simulink model "Microgrid_uniTLM_server"  (R2025b)
settings: Solver=ode3  StartTime=0.0  StopTime=1  FixedStep=params.sampleTime  RelTol=1e-3
InitFcn:
  | unitlmModelFile = get_param(bdroot, 'FileName');
  | if ~isempty(unitlmModelFile), addpath(fileparts(unitlmModelFile)); end
  | initialize_unitlm_microgrid();
  | clear unitlmModelFile
StartFcn:
  | unitlmModelFile = get_param(bdroot, 'FileName'); if ~isempty(unitlmModelFile), addpath(fileparts(unitlmModelFile)); end; try, if exist('unitlm_timing_probe', 'file') == 2, unitlm_timing_probe('start', 'server', bdroot); else, warning('uniTLM:TimingProbeNotFound', 'unitlm_timing_probe.m not found on MATLAB path; timing probe disabled.'); end; catch unitlmTimingError, warning('uniTLM:TimingProbeFailed', 'unitlm_timing_probe failed: %s', unitlmTimingError.message); end; clear unitlmModelFile
StopFcn:
  | unitlmModelFile = get_param(bdroot, 'FileName'); if ~isempty(unitlmModelFile), addpath(fileparts(unitlmModelFile)); end; try, if exist('unitlm_timing_probe', 'file') == 2, unitlm_timing_probe('stop', 'server', bdroot); else, warning('uniTLM:TimingProbeNotFound', 'unitlm_timing_probe.m not found on MATLAB path; timing probe disabled.'); end; catch unitlmTimingError, warning('uniTLM:TimingProbeFailed', 'unitlm_timing_probe failed: %s', unitlmTimingError.message); end; clear unitlmModelFile
  | %% StopFcn: save TLM server-side results
  | 
  | modelName = bdroot;
  | modelFile = get_param(modelName, 'FileName');
  | 
  | if isempty(modelFile)
  |     modelDir = pwd;
  | else
  |     modelDir = fileparts(modelFile);
  | end
  | 
  | resultDir = fullfile(modelDir, 'result');
  | 
  | if ~exist(resultDir, 'dir')
  |     mkdir(resultDir);
  | end
  | 
  | % Server-side workspace variables
  | variableNames = {
  |     'server_voltage'
  |     'server_current'
  |     'server_PQ'
  | };
  | 
  | serverTLMData = struct();
  | 
  | for k = 1:numel(variableNames)
  | 
  |     originalName = variableNames{k};
  |     saveName = [originalName, '_TLM'];
  | 
  |     if evalin('base', sprintf('exist(''%s'', ''var'')', originalName))
  |         serverTLMData.(saveName) = evalin('base', originalName);
  |     else
  |         warning( ...
  |             'StopFcn:MissingVariable', ...
  |             'Variable "%s" was not found in the base workspace.', ...
  |             originalName);
  |     end
  | end
  | 
  | % Save to result/server_TLM.mat
  | saveFile = fullfile(resultDir, 'server_TLM.mat');
  | save(saveFile, '-struct', 'serverTLMData');
  | 
  | fprintf('TLM server-side results saved to:\n%s\n', saveFile);
values from neighbouring files (symbols this model uses):
  Cf = Cf_pu*Cb    [initialize_unitlm_microgrid.m]
  f = logspace(log10(fMin), log10(fMax), nFrequency).'    [fit_non_heaviside_line_rational.m]    (also in initialize_unitlm_microgrid.m = 50)
  fsw1 = 10e3    (= 10000)    [initialize_unitlm_microgrid.m]
  Ip = 2*P/(3*Vp)    [initialize_unitlm_microgrid.m]
  L1 = L1_pu*Lb    [initialize_unitlm_microgrid.m]
  L2 = L2_pu*Lb    [initialize_unitlm_microgrid.m]
  L3 = L3_pu*Lb    [initialize_unitlm_microgrid.m]
  L4 = L4_pu*Lb    [initialize_unitlm_microgrid.m]
  Lc = Lc_pu*Lb    [initialize_unitlm_microgrid.m]
  Lf2 = Lf2_pu*Lb    [initialize_unitlm_microgrid.m]
  line_aHr = interface.line_aHr    [initialise_optimised_tlm_interface.m]    (also in initialize_unitlm_microgrid.m = real(line_aHr))
  line_aZc = interface.line_aZc    [initialise_optimised_tlm_interface.m]    (also in initialize_unitlm_microgrid.m = real(line_aZc))
  line_bHr = interface.line_bHr    [initialise_optimised_tlm_interface.m]    (also in initialize_unitlm_microgrid.m = real(line_bHr))
  line_bZc = interface.line_bZc    [initialise_optimised_tlm_interface.m]    (also in initialize_unitlm_microgrid.m = real(line_bZc))
  P = 5e6    (= 5000000)    [initialize_unitlm_microgrid.m]
  params = varargin{1}    [Client_co.m]    (also in Client_co_TLM.m; Server_co.m; Server_co_TLM.m; initialise_optimised_tlm_interface.m = config.cosimParams)
  R1 = R1_pu*Zb    [initialize_unitlm_microgrid.m]
  R2 = R2_pu*Zb    [initialize_unitlm_microgrid.m]
  R3 = R3_pu*Zb    [initialize_unitlm_microgrid.m]
  R4 = R4_pu*Zb    [initialize_unitlm_microgrid.m]
  Rdamp = Rf    [initialize_unitlm_microgrid.m]
  Rf = Rf_pu*Zb    [initialize_unitlm_microgrid.m]
  Rload1 = Vp/Ip    [initialize_unitlm_microgrid.m]
  Rload2 = Vp/Ip    [initialize_unitlm_microgrid.m]
  Rload3 = Vp/Ip    [initialize_unitlm_microgrid.m]
  Rv_pu = 0.1    [initialize_unitlm_microgrid.m]
  Sxfmr = 6.3e6    (= 6300000)    [initialize_unitlm_microgrid.m]
  Vac = sqrt(2)*Vline/sqrt(3)    [initialize_unitlm_microgrid.m]
  Vhv = 66e3    (= 66000)    [initialize_unitlm_microgrid.m]
  Vline = 690    [initialize_unitlm_microgrid.m]
  Vp = Vac    [initialize_unitlm_microgrid.m]
  Wb = 2*pi*f    (= 314.159265359)    [initialize_unitlm_microgrid.m]
  Xv_pu = 0.3    [initialize_unitlm_microgrid.m]
  Z_inf = interface.Z_inf    [initialise_optimised_tlm_interface.m]    (also in initialize_unitlm_microgrid.m = line_Zinf)
undefined symbols (not defined in the file or in its folder): DiscIntNeverNeededParam, DPL, dspblkCoreblockFVToolHelper, gcbh, Lline1
libraries: spsThreePhaseSeriesRLCBranchLib x14, spsControlledVoltageSourceLib x12, spsThreePhaseVIMeasurementLib x7, spsabctodq0Lib x6, slpidlib x4, spsThreePhaseBreakerLib x3, SimplusGT x3, spsThreePhaseTransformerTwoWindingsLib x3, spsPower3phInstantaneousLib x2, spsdq0toabcLib x2, spsDistributedParametersLineLib x1, simulink x1
(part 1 of 2)
settings Model: Creator=L  LastModifiedBy=Zhai Xinjie
settings DataIOCC: LimitDataPoints=on  SaveFormat=Array  ReturnWorkspaceOutputs=off
settings OptimizationCC: ReuseModelBlockBuffer=off  LifeSpan=inf
settings DebuggingCC: UnderspecifiedInitializationDetection=Classic  MergeDetectMultiDrivingBlocksExec=none  SolverPrmCheckMsg=warning  UnconnectedInputMsg=warning  UnconnectedOutputMsg=warning  UnconnectedLineMsg=warning  StateNameClashWarn=warning  SFUnexpectedBacktrackingDiag=warning  SFNoUnconditionalDefaultTransitionDiag=warning  SFExecutionAtInitializationDiag=none  ArithmeticOperatorsInVariantConditions=warning
settings HardwareCC: ProdBitPerPointer=32.0  ProdBitPerSizeT=32.0  ProdBitPerPtrDiffT=32.0  ProdLargestAtomicFloat=None  ProdIntDivRoundTo=Undefined  ProdEndianess=Unspecified  ProdWordSize=32.0  ProdHWDeviceType=32-bit Generic
settings ModelReferenceCC: EnableRefExpFcnMdlSchedulingChecks=on  PropagateSignalLabelsOutOfModel=off
settings SFSimCC: SimUseLocalCustomCode=off  CustomCodeUndefinedFunction=UseInterfaceOnly
settings RTWCC: RTWUseLocalCustomCode=off  GPUComputeCapability=3.5  DLArmComputeVersion=19.05
settings CodeAppCC: StateflowObjectComments=on
settings GRTTargetCC: TargetLangStandard=C89/C90 (ANSI)
settings ConfigComp: CovMetricSettings=dw  CovSaveCumulativeToWorkspaceVar=on  CovSaveSingleToWorkspaceVar=on  CovExternalEMLEnable=off
settings SimscapeCC: SimscapeNormalizeSystem=off

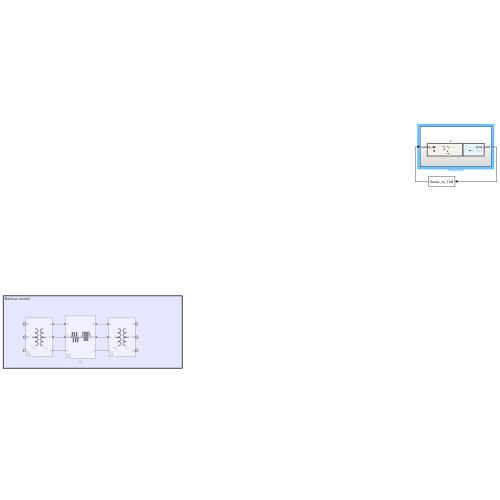
[thumbnail: Simulink's stored preview of the top-level diagram]
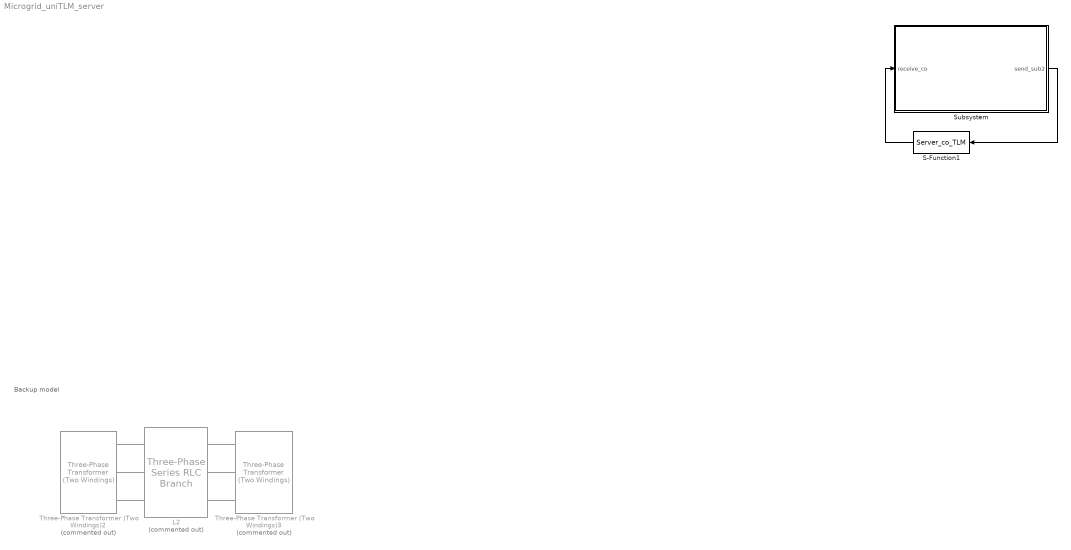
== system Microgrid_uniTLM_server ==
  note: Backup model
  L2 : spsThreePhaseSeriesRLCBranchLib/Three-Phase Series RLC Branch  Commented=on  LConnTagsString=A|B|C  RConnTagsString=A|B|C  BranchType=RL  Resistance=R2  Inductance=L2  Capacitance=1e-6  Measurements=None
  S-Function1 : S-Function  FunctionName=Server_co_TLM  SFunctionDeploymentMode=off  EnableBusSupport=off
  Subsystem : Subsystem
  Three-Phase Transformer (Two Windings)2 : spsThreePhaseTransformerTwoWindingsLib/Three-Phase Transformer (Two Windings)  Commented=on  Winding1Connection=Yg  Winding2Connection=Yg  CoreType=Three single-phase transformers  SetSaturation=off  Hysteresis=off  DataFile='hysteresis'  SetInitialFlux=off  Measurements=None  UNITS=pu  NominalPower=[ 250e6 , 50 ]  Winding1=[ 380e3 , 0.002 , 0.08 ]  Winding2=[ 33e3 , 0.002 , 0.08 ]  Rm=500  Lm=500  L0=0.5  Saturation=[ 0,0 ; 0.0024,1.2 ; 1.0,1.52 ]  InitialFluxes=[ 0.8 , -0.8 , 0.7 ]  BreakLoop=off  DiscreteSolver=Trapezoidal iterative  DataType=off  TransfoNumber=1
  Three-Phase Transformer (Two Windings)3 : spsThreePhaseTransformerTwoWindingsLib/Three-Phase Transformer (Two Windings)  Commented=on  Winding1Connection=Yg  Winding2Connection=Yg  CoreType=Three single-phase transformers  SetSaturation=off  Hysteresis=off  DataFile='hysteresis'  SetInitialFlux=off  Measurements=None  UNITS=pu  NominalPower=[ 250e6 , 50 ]  Winding1=[ 33e3 , 0.002 , 0.08 ]  Winding2=[ 380 , 0.002 , 0.08 ]  Rm=500  Lm=500  L0=0.5  Saturation=[ 0,0 ; 0.0024,1.2 ; 1.0,1.52 ]  InitialFluxes=[ 0.8 , -0.8 , 0.7 ]  BreakLoop=off  DiscreteSolver=Trapezoidal iterative  DataType=off  TransfoNumber=1
  wires:
  S-Function1/1 -> Subsystem/1(receive_co)
  Subsystem/1(send_sub2) -> S-Function1/1
  connections:
  Three-Phase Transformer (Two Windings)3/RConn1 -- L2/RConn1
  Three-Phase Transformer (Two Windings)3/RConn2 -- L2/RConn2
  Three-Phase Transformer (Two Windings)3/RConn3 -- L2/RConn3
  Three-Phase Transformer (Two Windings)2/RConn1 -- L2/LConn1
  Three-Phase Transformer (Two Windings)2/RConn2 -- L2/LConn2
  Three-Phase Transformer (Two Windings)2/RConn3 -- L2/LConn3

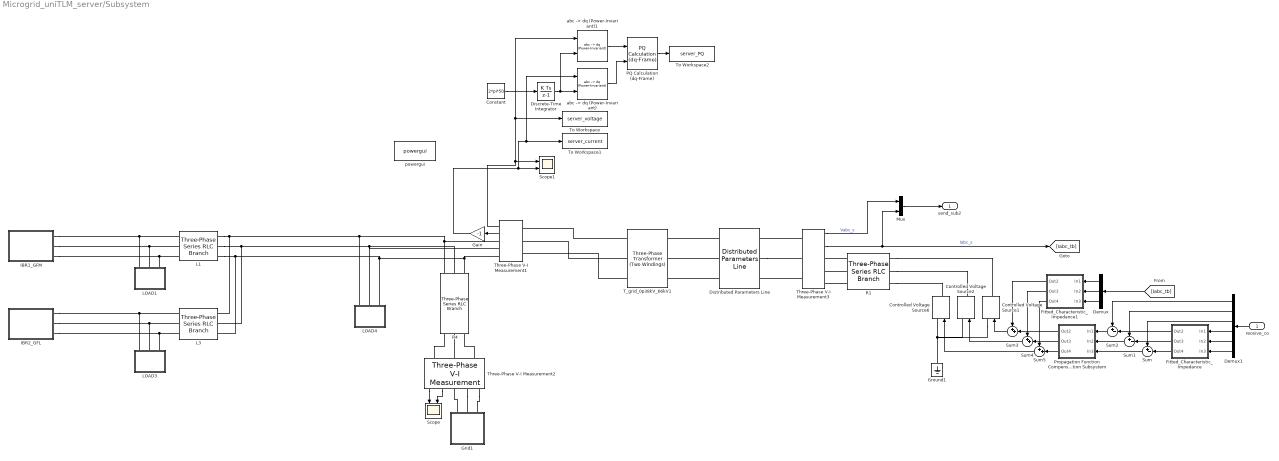
== system Microgrid_uniTLM_server/Subsystem ==
  receive_co : Inport
  Constant : Constant  Value=2*pi*50
  Controlled Voltage Source1 : spsControlledVoltageSourceLib/Controlled Voltage Source  Initialize=on  Source_Type=AC  Amplitude=0  Phase=0  Frequency=0  Measurements=None
  Controlled Voltage Source2 : spsControlledVoltageSourceLib/Controlled Voltage Source  Initialize=on  Source_Type=AC  Amplitude=0  Phase=0  Frequency=0  Measurements=None
  Controlled Voltage Source6 : spsControlledVoltageSourceLib/Controlled Voltage Source  Initialize=on  Source_Type=AC  Amplitude=0  Phase=0  Frequency=0  Measurements=None
  Demux : Demux  Outputs=3
  Demux1 : Demux  Outputs=6
  Discrete-Time Integrator : DiscreteIntegrator  SampleTime=-1  ICPrevOutput=DiscIntNeverNeededParam  ICPrevScaledInput=DiscIntNeverNeededParam
  Distributed Parameters Line : spsDistributedParametersLineLib/Distributed Parameters Line  Phases=3  Length=DPL.length  Frequency=DPL.freq  Resistance=DPL.R  Inductance=DPL.L  Capacitance=DPL.C  x1=[-0.0001175 0 0 0;-0.000117 0 0 0;-0.0001165 0 0 0;-0.000116 0 0 0;-0.0001155 0 0 0;-0.000115 0 0 0;-0.0001145 0 0 0;-0.000114 0 0 0;-0.0001135 0 0 0;-0.000113 0 0 0;-0.0001125 0 0 0;-0.000112 0 0 0;-0.0001115 0 0 0;-0.000111 0 0 0;-0.0001105 0 0 0;-0.00011 0 0 0;-0.0001095 0 0 0;-0.000109 0 0 0;-0.0001085 0 0 0;-0.000108 0 0 0;-0.0001075 0 0 0;-0.000107 0 0 0;-0.0001065 0 0 0;-0.000106 0 0 0;-0.0001055 0 0 0;-0.000105 0 0 0;-0.0001045 0 0 0;-0.000104 0 0 0;-0.0001035 0 0 0;-0.000103 0 0 0;-0.0001025 0 0 0;-0.000102 0 0 0;-0.0001015 0 0 0;-0.000101 0 0 0;-0.0001005 0 0 0;-0.0001 0 0 0;-9.95e-05 0 0 0;-9.9e-05 0 0 0;-9.85e-05 0 0 0;-9.8e-05 0 0 0;-9.75e-05 0 0 0;-9.7e-05 0 0 0;-9.65e-05 0 0 0;-9.6e-05 0 0 0;-9.55e-05 0 0 0;-9.5e-05 0 0 0;-9.45e-05 0 0 0;-9.4e-05 0 0 0;-9.35e-05 0 0 0;-9.3e-05 0 0 0;-9.25e-05 0 0 0;-9.2e-05 0 0 0;-9.15e-05 0 0 0;-9.1e-05 0 0 0;-9.05e-05 0 0 0;-9e-05 0 0 0;-8.95e-05 0 0 0;-8.9e-05 0 0 0;-8.85e-05 0 0 0;-8.8e-05 0 0 0;-8.75e-05 0 0 0;-8.7e-05 0 0 0;-8.65e-05 0 0 0;-8.6e-05 0 0 0;-8.55e-05 0 0 0;-8.5e-05 0 0 0;-8.45e-05 0 0 0;-8.4e-05 0 0 0;-8.35e-05 0 0 0;-8.3e-05 0 0 0;-8.25e-05 0 0 0;-8.2e-05 0 0 0;-8.15e-05 0 0 0;-8.1e-05 0 0 0;-8.05e-05 0 0 0;-8e-05 0 0 0;-7.95e-05 0 0 0;-7.9e-05 0 0 0;-7.85e-05 0 0 0;-7.8e-05 0 0 0;-7.75e-05 0 0 0;-7.7e-05 0 0 0;-7.65e-05 0 0 0;-7.6e-05 0 0 0;-7.55e-05 0 0 0;-7.5e-05 0 0 0;-7.45e-05 0 0 0;-7.4e-05 0 0 0;-7.35e-05 0 0 0;-7.3e-05 0 0 0;-7.25e-05 0 0 0;-7.2e-05 0 0 0;-7.15e-05 0 0 0;-7.1e-05 0 0 0;-7.05e-05 0 0 0;-7e-05 0 0 0;-6.95e-05 0 0 0;-6.9e-05 0 0 0;-6.85e-05 0 0 0;-6.8e-05 0 0 0;-6.75e-05 0 0 0;-6.7e-05 0 0 0;-6.65e-05 0 0 0;-6.6e-05 0 0 0;-6.55e-05 0 0 0;-6.5e-05 0 0 0;-6.45e-05 0 0 0;-6.4e-05 0 0 0;-6.35e-05 0 0 0;-6.3e-05 0 0 0;-6.25e-05 0 0 0;-6.2e-05 0 0 0;-6.15e-05 0 0 0;-6.1e-05 0 0 0;-6.05e-05 0 0 0;-6e-05 0 0 0;-5.95e-05 0 0 0;-5.9e-05 0 0 0;-5.85e-05 0 0 0;-5.8e-05 0 0 0;-5.75e-05 0 0 0;-5.7e-05 0 0 0;-5.65e-05 0 0 0;-5.6e-05 0 0 0;-5.55e-05 0 0 0;-5.5e-05 0 0 0;-5.45e-05 0 0 0;-5.4e-05 0 0 0;-5.35e-05 0 0 0;-5.3e-05 0 0 0;-5.25e-05 0 0 0;-5.2e-05 0 0 0;-5.15e-05 0 0 0;-5.1e-05 0 0 0;-5.05e-05 0 0 0;-5e-05 0 0 0;-4.95e-05 0 0 0;-4.9e-05 0 0 0;-4.85e-05 0 0 0;-4.8e-05 0 0 0;-4.75e-05 0 0 0;-4.7e-05 0 0 0;-4.65e-05 0 0 0;-4.6e-05 0 0 0;-4.55e-05 0 0 0;-4.5e-05 0 0 0;-4.45e-05 0 0 0;-4.4e-05 0 0 0;-4.35e-05 0 0 0;-4.3e-05 0 0 0;-4.25e-05 0 0 0;-4.2e-05 0 0 0;-4.15e-05 0 0 0;-4.1e-05 0 0 0;-4.05e-05 0 0 0;-4e-05 0 0 0;-3.95e-05 0 0 0;-3.9e-05 0 0 0;-3.85e-05 0 0 0;-3.8e-05 0 0 0;-3.75e-05 0 0 0;-3.7e-05 0 0 0;-3.65e-05 0 0 0;-3.6e-05 0 0 0;-3.55e-05 0 0 0;-3.5e-05 0 0 0;-3.45e-05 0 0 0;-3.4e-05 0 0 0;-3.35e-05 0 0 0;-3.3e-05 0 0 0;-3.25e-05 0 0 0;-3.2e-05 0 0 0;-3.15e-05 0 0 0;-3.1e-05 0 0 0;-3.05e-05 0 0 0;-3e-05 0 0 0;-2.95e-05 0 0 0;-2.9e-05 0 0 0;-2.85e-05 0 0 0;-2.8e-05 0 0 0;-2.75e-05 0 0 0;-2.7e-05 0 0 0;-2.65e-05 0 0 0;-2.6e-05 0 0 0;-2.55e-05 0 0 0;-2.5e-05 0 0 0;-2.45e-05 0 0 0;-2.4e-05 0 0 0;-2.35e-05 0 0 0;-2.3e-05 0 0 0;-2.25e-05 0 0 0;-2.2e-05 0 0 0;-2.15e-05 0 0 0;-2.1e-05 0 0 0;-2.05e-05 0 0 0;-2e-05 0 0 0;-1.95e-05 0 0 0;-1.9e-05 0 0 0;-1.85e-05 0 0 0;-1.8e-05 0 0 0;-1.75e-05 0 0 0;-1.7e-05 0 0 0;-1.65e-05 0 0 0;-1.6e-05 0 0 0;-1.55e-05 0 0 0;-1.5e-05 0 0 0;-1.45e-05 0 0 0;-1.4e-05 0 0 0;-1.35e-05 0 0 0;-1.3e-05 0 0 0;-1.25e-05 0 0 0;-1.2e-05 0 0 0;-1.15e-05 0 0 0;-1.1e-05 0 0 0;-1.05e-05 0 0 0;-1e-05 0 0 0;-9.5e-06 0 0 0;-9e-06 0 0 0;-8.5e-06 0 0 0;-8e-06 0 0 0;-7.5e-06 0 0 0;-7e-06 0 0 0;-6.5e-06 0 0 0;-6e-06 0 0 0;-5.5e-06 0 0 0;-5e-06 0 0 0;-4.5e-06 0 0 0;-4e-06 0 0 0;-3.5e-06 0 0 0;-3e-06 0 0 0;-2.5e-06 0 0 0;-2e-06 0 0 0;-1.5e-06 0 0 0;-1e-06 0 0 0;-5e-07 0 0 0]  x2=[-0.0001175 0 0 0;-0.000117 0 0 0;-0.0001165 0 0 0;-0.000116 0 0 0;-0.0001155 0 0 0;-0.000115 0 0 0;-0.0001145 0 0 0;-0.000114 0 0 0;-0.0001135 0 0 0;-0.000113 0 0 0;-0.0001125 0 0 0;-0.000112 0 0 0;-0.0001115 0 0 0;-0.000111 0 0 0;-0.0001105 0 0 0;-0.00011 0 0 0;-0.0001095 0 0 0;-0.000109 0 0 0;-0.0001085 0 0 0;-0.000108 0 0 0;-0.0001075 0 0 0;-0.000107 0 0 0;-0.0001065 0 0 0;-0.000106 0 0 0;-0.0001055 0 0 0;-0.000105 0 0 0;-0.0001045 0 0 0;-0.000104 0 0 0;-0.0001035 0 0 0;-0.000103 0 0 0;-0.0001025 0 0 0;-0.000102 0 0 0;-0.0001015 0 0 0;-0.000101 0 0 0;-0.0001005 0 0 0;-0.0001 0 0 0;-9.95e-05 0 0 0;-9.9e-05 0 0 0;-9.85e-05 0 0 0;-9.8e-05 0 0 0;-9.75e-05 0 0 0;-9.7e-05 0 0 0;-9.65e-05 0 0 0;-9.6e-05 0 0 0;-9.55e-05 0 0 0;-9.5e-05 0 0 0;-9.45e-05 0 0 0;-9.4e-05 0 0 0;-9.35e-05 0 0 0;-9.3e-05 0 0 0;-9.25e-05 0 0 0;-9.2e-05 0 0 0;-9.15e-05 0 0 0;-9.1e-05 0 0 0;-9.05e-05 0 0 0;-9e-05 0 0 0;-8.95e-05 0 0 0;-8.9e-05 0 0 0;-8.85e-05 0 0 0;-8.8e-05 0 0 0;-8.75e-05 0 0 0;-8.7e-05 0 0 0;-8.65e-05 0 0 0;-8.6e-05 0 0 0;-8.55e-05 0 0 0;-8.5e-05 0 0 0;-8.45e-05 0 0 0;-8.4e-05 0 0 0;-8.35e-05 0 0 0;-8.3e-05 0 0 0;-8.25e-05 0 0 0;-8.2e-05 0 0 0;-8.15e-05 0 0 0;-8.1e-05 0 0 0;-8.05e-05 0 0 0;-8e-05 0 0 0;-7.95e-05 0 0 0;-7.9e-05 0 0 0;-7.85e-05 0 0 0;-7.8e-05 0 0 0;-7.75e-05 0 0 0;-7.7e-05 0 0 0;-7.65e-05 0 0 0;-7.6e-05 0 0 0;-7.55e-05 0 0 0;-7.5e-05 0 0 0;-7.45e-05 0 0 0;-7.4e-05 0 0 0;-7.35e-05 0 0 0;-7.3e-05 0 0 0;-7.25e-05 0 0 0;-7.2e-05 0 0 0;-7.15e-05 0 0 0;-7.1e-05 0 0 0;-7.05e-05 0 0 0;-7e-05 0 0 0;-6.95e-05 0 0 0;-6.9e-05 0 0 0;-6.85e-05 0 0 0;-6.8e-05 0 0 0;-6.75e-05 0 0 0;-6.7e-05 0 0 0;-6.65e-05 0 0 0;-6.6e-05 0 0 0;-6.55e-05 0 0 0;-6.5e-05 0 0 0;-6.45e-05 0 0 0;-6.4e-05 0 0 0;-6.35e-05 0 0 0;-6.3e-05 0 0 0;-6.25e-05 0 0 0;-6.2e-05 0 0 0;-6.15e-05 0 0 0;-6.1e-05 0 0 0;-6.05e-05 0 0 0;-6e-05 0 0 0;-5.95e-05 0 0 0;-5.9e-05 0 0 0;-5.85e-05 0 0 0;-5.8e-05 0 0 0;-5.75e-05 0 0 0;-5.7e-05 0 0 0;-5.65e-05 0 0 0;-5.6e-05 0 0 0;-5.55e-05 0 0 0;-5.5e-05 0 0 0;-5.45e-05 0 0 0;-5.4e-05 0 0 0;-5.35e-05 0 0 0;-5.3e-05 0 0 0;-5.25e-05 0 0 0;-5.2e-05 0 0 0;-5.15e-05 0 0 0;-5.1e-05 0 0 0;-5.05e-05 0 0 0;-5e-05 0 0 0;-4.95e-05 0 0 0;-4.9e-05 0 0 0;-4.85e-05 0 0 0;-4.8e-05 0 0 0;-4.75e-05 0 0 0;-4.7e-05 0 0 0;-4.65e-05 0 0 0;-4.6e-05 0 0 0;-4.55e-05 0 0 0;-4.5e-05 0 0 0;-4.45e-05 0 0 0;-4.4e-05 0 0 0;-4.35e-05 0 0 0;-4.3e-05 0 0 0;-4.25e-05 0 0 0;-4.2e-05 0 0 0;-4.15e-05 0 0 0;-4.1e-05 0 0 0;-4.05e-05 0 0 0;-4e-05 0 0 0;-3.95e-05 0 0 0;-3.9e-05 0 0 0;-3.85e-05 0 0 0;-3.8e-05 0 0 0;-3.75e-05 0 0 0;-3.7e-05 0 0 0;-3.65e-05 0 0 0;-3.6e-05 0 0 0;-3.55e-05 0 0 0;-3.5e-05 0 0 0;-3.45e-05 0 0 0;-3.4e-05 0 0 0;-3.35e-05 0 0 0;-3.3e-05 0 0 0;-3.25e-05 0 0 0;-3.2e-05 0 0 0;-3.15e-05 0 0 0;-3.1e-05 0 0 0;-3.05e-05 0 0 0;-3e-05 0 0 0;-2.95e-05 0 0 0;-2.9e-05 0 0 0;-2.85e-05 0 0 0;-2.8e-05 0 0 0;-2.75e-05 0 0 0;-2.7e-05 0 0 0;-2.65e-05 0 0 0;-2.6e-05 0 0 0;-2.55e-05 0 0 0;-2.5e-05 0 0 0;-2.45e-05 0 0 0;-2.4e-05 0 0 0;-2.35e-05 0 0 0;-2.3e-05 0 0 0;-2.25e-05 0 0 0;-2.2e-05 0 0 0;-2.15e-05 0 0 0;-2.1e-05 0 0 0;-2.05e-05 0 0 0;-2e-05 0 0 0;-1.95e-05 0 0 0;-1.9e-05 0 0 0;-1.85e-05 0 0 0;-1.8e-05 0 0 0;-1.75e-05 0 0 0;-1.7e-05 0 0 0;-1.65e-05 0 0 0;-1.6e-05 0 0 0;-1.55e-05 0 0 0;-1.5e-05 0 0 0;-1.45e-05 0 0 0;-1.4e-05 0 0 0;-1.35e-05 0 0 0;-1.3e-05 0 0 0;-1.25e-05 0 0 0;-1.2e-05 0 0 0;-1.15e-05 0 0 0;-1.1e-05 0 0 0;-1.05e-05 0 0 0;-1e-05 0 0 0;-9.5e-06 0 0 0;-9e-06 0 0 0;-8.5e-06 0 0 0;-8e-06 0 0 0;-7.5e-06 0 0 0;-7e-06 0 0 0;-6.5e-06 0 0 0;-6e-06 0 0 0;-5.5e-06 0 0 0;-5e-06 0 0 0;-4.5e-06 0 0 0;-4e-06 0 0 0;-3.5e-06 0 0 0;-3e-06 0 0 0;-2.5e-06 0 0 0;-2e-06 0 0 0;-1.5e-06 0 0 0;-1e-06 0 0 0;-5e-07 0 0 0]  x3=[-0.0001175 0 0 0;-0.000117 0 0 0;-0.0001165 0 0 0;-0.000116 0 0 0;-0.0001155 0 0 0;-0.000115 0 0 0;-0.0001145 0 0 0;-0.000114 0 0 0;-0.0001135 0 0 0;-0.000113 0 0 0;-0.0001125 0 0 0;-0.000112 0 0 0;-0.0001115 0 0 0;-0.000111 0 0 0;-0.0001105 0 0 0;-0.00011 0 0 0;-0.0001095 0 0 0;-0.000109 0 0 0;-0.0001085 0 0 0;-0.000108 0 0 0;-0.0001075 0 0 0;-0.000107 0 0 0;-0.0001065 0 0 0;-0.000106 0 0 0;-0.0001055 0 0 0;-0.000105 0 0 0;-0.0001045 0 0 0;-0.000104 0 0 0;-0.0001035 0 0 0;-0.000103 0 0 0;-0.0001025 0 0 0;-0.000102 0 0 0;-0.0001015 0 0 0;-0.000101 0 0 0;-0.0001005 0 0 0;-0.0001 0 0 0;-9.95e-05 0 0 0;-9.9e-05 0 0 0;-9.85e-05 0 0 0;-9.8e-05 0 0 0;-9.75e-05 0 0 0;-9.7e-05 0 0 0;-9.65e-05 0 0 0;-9.6e-05 0 0 0;-9.55e-05 0 0 0;-9.5e-05 0 0 0;-9.45e-05 0 0 0;-9.4e-05 0 0 0;-9.35e-05 0 0 0;-9.3e-05 0 0 0;-9.25e-05 0 0 0;-9.2e-05 0 0 0;-9.15e-05 0 0 0;-9.1e-05 0 0 0;-9.05e-05 0 0 0;-9e-05 0 0 0;-8.95e-05 0 0 0;-8.9e-05 0 0 0;-8.85e-05 0 0 0;-8.8e-05 0 0 0;-8.75e-05 0 0 0;-8.7e-05 0 0 0;-8.65e-05 0 0 0;-8.6e-05 0 0 0;-8.55e-05 0 0 0;-8.5e-05 0 0 0;-8.45e-05 0 0 0;-8.4e-05 0 0 0;-8.35e-05 0 0 0;-8.3e-05 0 0 0;-8.25e-05 0 0 0;-8.2e-05 0 0 0;-8.15e-05 0 0 0;-8.1e-05 0 0 0;-8.05e-05 0 0 0;-8e-05 0 0 0;-7.95e-05 0 0 0;-7.9e-05 0 0 0;-7.85e-05 0 0 0;-7.8e-05 0 0 0;-7.75e-05 0 0 0;-7.7e-05 0 0 0;-7.65e-05 0 0 0;-7.6e-05 0 0 0;-7.55e-05 0 0 0;-7.5e-05 0 0 0;-7.45e-05 0 0 0;-7.4e-05 0 0 0;-7.35e-05 0 0 0;-7.3e-05 0 0 0;-7.25e-05 0 0 0;-7.2e-05 0 0 0;-7.15e-05 0 0 0;-7.1e-05 0 0 0;-7.05e-05 0 0 0;-7e-05 0 0 0;-6.95e-05 0 0 0;-6.9e-05 0 0 0;-6.85e-05 0 0 0;-6.8e-05 0 0 0;-6.75e-05 0 0 0;-6.7e-05 0 0 0;-6.65e-05 0 0 0;-6.6e-05 0 0 0;-6.55e-05 0 0 0;-6.5e-05 0 0 0;-6.45e-05 0 0 0;-6.4e-05 0 0 0;-6.35e-05 0 0 0;-6.3e-05 0 0 0;-6.25e-05 0 0 0;-6.2e-05 0 0 0;-6.15e-05 0 0 0;-6.1e-05 0 0 0;-6.05e-05 0 0 0;-6e-05 0 0 0;-5.95e-05 0 0 0;-5.9e-05 0 0 0;-5.85e-05 0 0 0;-5.8e-05 0 0 0;-5.75e-05 0 0 0;-5.7e-05 0 0 0;-5.65e-05 0 0 0;-5.6e-05 0 0 0;-5.55e-05 0 0 0;-5.5e-05 0 0 0;-5.45e-05 0 0 0;-5.4e-05 0 0 0;-5.35e-05 0 0 0;-5.3e-05 0 0 0;-5.25e-05 0 0 0;-5.2e-05 0 0 0;-5.15e-05 0 0 0;-5.1e-05 0 0 0;-5.05e-05 0 0 0;-5e-05 0 0 0;-4.95e-05 0 0 0;-4.9e-05 0 0 0;-4.85e-05 0 0 0;-4.8e-05 0 0 0;-4.75e-05 0 0 0;-4.7e-05 0 0 0;-4.65e-05 0 0 0;-4.6e-05 0 0 0;-4.55e-05 0 0 0;-4.5e-05 0 0 0;-4.45e-05 0 0 0;-4.4e-05 0 0 0;-4.35e-05 0 0 0;-4.3e-05 0 0 0;-4.25e-05 0 0 0;-4.2e-05 0 0 0;-4.15e-05 0 0 0;-4.1e-05 0 0 0;-4.05e-05 0 0 0;-4e-05 0 0 0;-3.95e-05 0 0 0;-3.9e-05 0 0 0;-3.85e-05 0 0 0;-3.8e-05 0 0 0;-3.75e-05 0 0 0;-3.7e-05 0 0 0;-3.65e-05 0 0 0;-3.6e-05 0 0 0;-3.55e-05 0 0 0;-3.5e-05 0 0 0;-3.45e-05 0 0 0;-3.4e-05 0 0 0;-3.35e-05 0 0 0;-3.3e-05 0 0 0;-3.25e-05 0 0 0;-3.2e-05 0 0 0;-3.15e-05 0 0 0;-3.1e-05 0 0 0;-3.05e-05 0 0 0;-3e-05 0 0 0;-2.95e-05 0 0 0;-2.9e-05 0 0 0;-2.85e-05 0 0 0;-2.8e-05 0 0 0;-2.75e-05 0 0 0;-2.7e-05 0 0 0;-2.65e-05 0 0 0;-2.6e-05 0 0 0;-2.55e-05 0 0 0;-2.5e-05 0 0 0;-2.45e-05 0 0 0;-2.4e-05 0 0 0;-2.35e-05 0 0 0;-2.3e-05 0 0 0;-2.25e-05 0 0 0;-2.2e-05 0 0 0;-2.15e-05 0 0 0;-2.1e-05 0 0 0;-2.05e-05 0 0 0;-2e-05 0 0 0;-1.95e-05 0 0 0;-1.9e-05 0 0 0;-1.85e-05 0 0 0;-1.8e-05 0 0 0;-1.75e-05 0 0 0;-1.7e-05 0 0 0;-1.65e-05 0 0 0;-1.6e-05 0 0 0;-1.55e-05 0 0 0;-1.5e-05 0 0 0;-1.45e-05 0 0 0;-1.4e-05 0 0 0;-1.35e-05 0 0 0;-1.3e-05 0 0 0;-1.25e-05 0 0 0;-1.2e-05 0 0 0;-1.15e-05 0 0 0;-1.1e-05 0 0 0;-1.05e-05 0 0 0;-1e-05 0 0 0;-9.5e-06 0 0 0;-9e-06 0 0 0;-8.5e-06 0 0 0;-8e-06 0 0 0;-7.5e-06 0 0 0;-7e-06 0 0 0;-6.5e-06 0 0 0;-6e-06 0 0 0;-5.5e-06 0 0 0;-5e-06 0 0 0;-4.5e-06 0 0 0;-4e-06 0 0 0;-3.5e-06 0 0 0;-3e-06 0 0 0;-2.5e-06 0 0 0;-2e-06 0 0 0;-1.5e-06 0 0 0;-1e-06 0 0 0;-5e-07 0 0 0]  x4=[-0.0001175 0 0 0;-0.000117 0 0 0;-0.0001165 0 0 0;-0.000116 0 0 0;-0.0001155 0 0 0;-0.000115 0 0 0;-0.0001145 0 0 0;-0.000114 0 0 0;-0.0001135 0 0 0;-0.000113 0 0 0;-0.0001125 0 0 0;-0.000112 0 0 0;-0.0001115 0 0 0;-0.000111 0 0 0;-0.0001105 0 0 0;-0.00011 0 0 0;-0.0001095 0 0 0;-0.000109 0 0 0;-0.0001085 0 0 0;-0.000108 0 0 0;-0.0001075 0 0 0;-0.000107 0 0 0;-0.0001065 0 0 0;-0.000106 0 0 0;-0.0001055 0 0 0;-0.000105 0 0 0;-0.0001045 0 0 0;-0.000104 0 0 0;-0.0001035 0 0 0;-0.000103 0 0 0;-0.0001025 0 0 0;-0.000102 0 0 0;-0.0001015 0 0 0;-0.000101 0 0 0;-0.0001005 0 0 0;-0.0001 0 0 0;-9.95e-05 0 0 0;-9.9e-05 0 0 0;-9.85e-05 0 0 0;-9.8e-05 0 0 0;-9.75e-05 0 0 0;-9.7e-05 0 0 0;-9.65e-05 0 0 0;-9.6e-05 0 0 0;-9.55e-05 0 0 0;-9.5e-05 0 0 0;-9.45e-05 0 0 0;-9.4e-05 0 0 0;-9.35e-05 0 0 0;-9.3e-05 0 0 0;-9.25e-05 0 0 0;-9.2e-05 0 0 0;-9.15e-05 0 0 0;-9.1e-05 0 0 0;-9.05e-05 0 0 0;-9e-05 0 0 0;-8.95e-05 0 0 0;-8.9e-05 0 0 0;-8.85e-05 0 0 0;-8.8e-05 0 0 0;-8.75e-05 0 0 0;-8.7e-05 0 0 0;-8.65e-05 0 0 0;-8.6e-05 0 0 0;-8.55e-05 0 0 0;-8.5e-05 0 0 0;-8.45e-05 0 0 0;-8.4e-05 0 0 0;-8.35e-05 0 0 0;-8.3e-05 0 0 0;-8.25e-05 0 0 0;-8.2e-05 0 0 0;-8.15e-05 0 0 0;-8.1e-05 0 0 0;-8.05e-05 0 0 0;-8e-05 0 0 0;-7.95e-05 0 0 0;-7.9e-05 0 0 0;-7.85e-05 0 0 0;-7.8e-05 0 0 0;-7.75e-05 0 0 0;-7.7e-05 0 0 0;-7.65e-05 0 0 0;-7.6e-05 0 0 0;-7.55e-05 0 0 0;-7.5e-05 0 0 0;-7.45e-05 0 0 0;-7.4e-05 0 0 0;-7.35e-05 0 0 0;-7.3e-05 0 0 0;-7.25e-05 0 0 0;-7.2e-05 0 0 0;-7.15e-05 0 0 0;-7.1e-05 0 0 0;-7.05e-05 0 0 0;-7e-05 0 0 0;-6.95e-05 0 0 0;-6.9e-05 0 0 0;-6.85e-05 0 0 0;-6.8e-05 0 0 0;-6.75e-05 0 0 0;-6.7e-05 0 0 0;-6.65e-05 0 0 0;-6.6e-05 0 0 0;-6.55e-05 0 0 0;-6.5e-05 0 0 0;-6.45e-05 0 0 0;-6.4e-05 0 0 0;-6.35e-05 0 0 0;-6.3e-05 0 0 0;-6.25e-05 0 0 0;-6.2e-05 0 0 0;-6.15e-05 0 0 0;-6.1e-05 0 0 0;-6.05e-05 0 0 0;-6e-05 0 0 0;-5.95e-05 0 0 0;-5.9e-05 0 0 0;-5.85e-05 0 0 0;-5.8e-05 0 0 0;-5.75e-05 0 0 0;-5.7e-05 0 0 0;-5.65e-05 0 0 0;-5.6e-05 0 0 0;-5.55e-05 0 0 0;-5.5e-05 0 0 0;-5.45e-05 0 0 0;-5.4e-05 0 0 0;-5.35e-05 0 0 0;-5.3e-05 0 0 0;-5.25e-05 0 0 0;-5.2e-05 0 0 0;-5.15e-05 0 0 0;-5.1e-05 0 0 0;-5.05e-05 0 0 0;-5e-05 0 0 0;-4.95e-05 0 0 0;-4.9e-05 0 0 0;-4.85e-05 0 0 0;-4.8e-05 0 0 0;-4.75e-05 0 0 0;-4.7e-05 0 0 0;-4.65e-05 0 0 0;-4.6e-05 0 0 0;-4.55e-05 0 0 0;-4.5e-05 0 0 0;-4.45e-05 0 0 0;-4.4e-05 0 0 0;-4.35e-05 0 0 0;-4.3e-05 0 0 0;-4.25e-05 0 0 0;-4.2e-05 0 0 0;-4.15e-05 0 0 0;-4.1e-05 0 0 0;-4.05e-05 0 0 0;-4e-05 0 0 0;-3.95e-05 0 0 0;-3.9e-05 0 0 0;-3.85e-05 0 0 0;-3.8e-05 0 0 0;-3.75e-05 0 0 0;-3.7e-05 0 0 0;-3.65e-05 0 0 0;-3.6e-05 0 0 0;-3.55e-05 0 0 0;-3.5e-05 0 0 0;-3.45e-05 0 0 0;-3.4e-05 0 0 0;-3.35e-05 0 0 0;-3.3e-05 0 0 0;-3.25e-05 0 0 0;-3.2e-05 0 0 0;-3.15e-05 0 0 0;-3.1e-05 0 0 0;-3.05e-05 0 0 0;-3e-05 0 0 0;-2.95e-05 0 0 0;-2.9e-05 0 0 0;-2.85e-05 0 0 0;-2.8e-05 0 0 0;-2.75e-05 0 0 0;-2.7e-05 0 0 0;-2.65e-05 0 0 0;-2.6e-05 0 0 0;-2.55e-05 0 0 0;-2.5e-05 0 0 0;-2.45e-05 0 0 0;-2.4e-05 0 0 0;-2.35e-05 0 0 0;-2.3e-05 0 0 0;-2.25e-05 0 0 0;-2.2e-05 0 0 0;-2.15e-05 0 0 0;-2.1e-05 0 0 0;-2.05e-05 0 0 0;-2e-05 0 0 0;-1.95e-05 0 0 0;-1.9e-05 0 0 0;-1.85e-05 0 0 0;-1.8e-05 0 0 0;-1.75e-05 0 0 0;-1.7e-05 0 0 0;-1.65e-05 0 0 0;-1.6e-05 0 0 0;-1.55e-05 0 0 0;-1.5e-05 0 0 0;-1.45e-05 0 0 0;-1.4e-05 0 0 0;-1.35e-05 0 0 0;-1.3e-05 0 0 0;-1.25e-05 0 0 0;-1.2e-05 0 0 0;-1.15e-05 0 0 0;-1.1e-05 0 0 0;-1.05e-05 0 0 0;-1e-05 0 0 0;-9.5e-06 0 0 0;-9e-06 0 0 0;-8.5e-06 0 0 0;-8e-06 0 0 0;-7.5e-06 0 0 0;-7e-06 0 0 0;-6.5e-06 0 0 0;-6e-06 0 0 0;-5.5e-06 0 0 0;-5e-06 0 0 0;-4.5e-06 0 0 0;-4e-06 0 0 0;-3.5e-06 0 0 0;-3e-06 0 0 0;-2.5e-06 0 0 0;-2e-06 0 0 0;-1.5e-06 0 0 0;-1e-06 0 0 0;-5e-07 0 0 0]  x5=0.000117250613940415  V1=ones(3,3)  V2=ones(3,3)  I1=ones(3,3)  I2=ones(3,3)  nHarmo=1  Measurements=None  Decoupling=off  VsMag0=0  VrMag0=0  VsAngle0=0  VrAngle0=0  IsMag0=0  IrMag0=0  IsAngle0=0  IrAngle0=0
      settings: LibrarySourceBlock=sps_lib/Power Grid Elements/Distributed Parameters Line
  Fitted_Characteristic_Impedance : Subsystem
  Fitted_Characteristic_Impedance1 : Subsystem
  Gain : Gain  Gain=-1
  Grid1 : Subsystem
  Ground1 : spsGroundLib/Ground  LConnTagsString=a
  IBR1_GFM : Subsystem
  IBR2_GFL : Subsystem
  L1 : spsThreePhaseSeriesRLCBranchLib/Three-Phase Series RLC Branch  LConnTagsString=A|B|C  RConnTagsString=A|B|C  BranchType=RL  Resistance=R1  Inductance=L1  Capacitance=1e-6  Measurements=None
  L3 : spsThreePhaseSeriesRLCBranchLib/Three-Phase Series RLC Branch  LConnTagsString=A|B|C  RConnTagsString=A|B|C  BranchType=RL  Resistance=R3  Inductance=L3  Capacitance=1e-6  Measurements=None
  LOAD1 : Subsystem
  LOAD3 : Subsystem
  LOAD4 : Subsystem
  Mux : Mux  Inputs=2
  PQ Calculation (dq-Frame) : SimplusGT/PQ Calculation (dq-Frame)  SystemSampleTime=-1  VariantActivationTime=update diagram  EmptyChoice=off  PassThrough=off  PassThroughVariantControl=(default)  EmptyChoiceVariantControl=(default)  AllowFlexibleInterface=on  Latency=0  AutoFrameSizeCalculation=off
      settings: SourceProductName=Simplus Grid Tool
  Propagation Function Compensation Subsystem : Subsystem
  R1 : spsThreePhaseSeriesRLCBranchLib/Three-Phase Series RLC Branch  LConnTagsString=A|B|C  RConnTagsString=A|B|C  BranchType=R  Resistance=Z_inf  Inductance=L4  Capacitance=1e-6  Measurements=None
  R4 : spsThreePhaseSeriesRLCBranchLib/Three-Phase Series RLC Branch  LConnTagsString=A|B|C  RConnTagsString=A|B|C  BranchType=RL  Resistance=R4  Inductance=L4  Capacitance=1e-6  Measurements=None
  Scope : Scope  NumInputPorts=2
      settings: ActiveDisplayYMinimum=-671.75144212722125  ActiveDisplayYMaximum=671.75144212722125
  Scope1 : Scope  NumInputPorts=2
      settings: ActiveDisplayYMinimum=-1224.8177993461568  ActiveDisplayYMaximum=1227.6312431891313  DataLoggingVariableName=ScopeData2
  Sum : Sum  Inputs=+-|
  Sum1 : Sum  Inputs=+-|
  Sum2 : Sum  Inputs=+-|
  Sum3 : Sum  Inputs=++|
  Sum4 : Sum  Inputs=++|
  Sum5 : Sum  Inputs=++|
  T_grid_0p38kV_66kV1 : spsThreePhaseTransformerTwoWindingsLib/Three-Phase Transformer (Two Windings)  Winding1Connection=Yg  Winding2Connection=Yg  CoreType=Three single-phase transformers  SetSaturation=off  Hysteresis=off  DataFile='hysteresis'  SetInitialFlux=off  Measurements=None  UNITS=pu  NominalPower=[Sxfmr, f]  Winding1=[Vhv, 0.002, 0.04]  Winding2=[Vline, 0.002, 0.04]  Rm=500  Lm=500  L0=0.5  Saturation=[ 0,0 ; 0.0024,1.2 ; 1.0,1.52 ]  InitialFluxes=[ 0.8 , -0.8 , 0.7 ]  BreakLoop=off  DiscreteSolver=Trapezoidal iterative  DataType=off  TransfoNumber=1
  Three-Phase V-I Measurement1 : spsThreePhaseVIMeasurementLib/Three-Phase V-I Measurement  VoltageMeasurement=phase-to-phase  SetLabelV=off  LabelV=Vabc1  Vpu=off  VpuLL=off  CurrentMeasurement=yes  SetLabelI=off  LabelI=Iabc3  Ipu=off  Pbase=100e6  Vbase=500e3  OutputType=Complex  PhasorSimulation=off  PSBequivalent=0
  Three-Phase V-I Measurement2 : spsThreePhaseVIMeasurementLib/Three-Phase V-I Measurement  VoltageMeasurement=phase-to-phase  SetLabelV=off  LabelV=Vabc1  Vpu=off  VpuLL=off  CurrentMeasurement=yes  SetLabelI=off  LabelI=Iabc3  Ipu=off  Pbase=100e6  Vbase=500e3  OutputType=Complex  PhasorSimulation=off  PSBequivalent=0
  Three-Phase V-I Measurement3 : spsThreePhaseVIMeasurementLib/Three-Phase V-I Measurement  VoltageMeasurement=phase-to-ground  SetLabelV=off  LabelV=Vabc_s  Vpu=off  VpuLL=off  CurrentMeasurement=yes  SetLabelI=off  LabelI=Iabc_s  Ipu=off  Pbase=100e6  Vbase=500e3  OutputType=Complex  PhasorSimulation=off  PSBequivalent=0
  To Workspace : ToWorkspace  VariableName=server_voltage  SaveFormat=Timeseries  SampleTime=-1
  To Workspace1 : ToWorkspace  VariableName=server_current  SaveFormat=Timeseries  SampleTime=-1
  To Workspace2 : ToWorkspace  VariableName=server_PQ  SaveFormat=Timeseries  SampleTime=-1
  "abc -> dq (Power-Invariant)" : SimplusGT/abc -> dq (Power-Invariant)  SystemSampleTime=-1  VariantActivationTime=update diagram  EmptyChoice=off  PassThrough=off  PassThroughVariantControl=(default)  EmptyChoiceVariantControl=(default)  AllowFlexibleInterface=on  Latency=0  AutoFrameSizeCalculation=off
      settings: SourceProductName=Simplus Grid Tool
  "abc -> dq (Power-Invariant)1" : SimplusGT/abc -> dq (Power-Invariant)  SystemSampleTime=-1  VariantActivationTime=update diagram  EmptyChoice=off  PassThrough=off  PassThroughVariantControl=(default)  EmptyChoiceVariantControl=(default)  AllowFlexibleInterface=on  Latency=0  AutoFrameSizeCalculation=off
      settings: SourceProductName=Simplus Grid Tool
  powergui : spspowerguiLib/powergui  Priority=1  SimulationMode=Discrete  SampleTime=params.sampleTime  frequency=60  Iterations=50  frequencyindice=0  Pbase=100e6  ErrMax=1e-4  UnitsV=kV  UnitsW=MW  buscounter=0  FunctionMessages=off  echomessages=off  EnableUseOfTLC=off  CurrentSourceSwitches=off  DisableSnubberDevices=off  DisableRonSwitches=off  DisableVfSwitches=off  DisplayEquations=off  AutomaticDiscreteSolvers=off  SolverType=Tustin/Backward Euler (TBE)  Interpol=off  ExternalGateDelay=off  methode=off  Ts=100  x0status=blocks  SPID=on  SwTol=0  HookPort=off  NonlinearTolerance=1e-4  nMaxIteration=100  ContinueOnMaxIteration=off  RestoreLinks=warning  ResistiveCurrentMeasurement=off  Frange=[0:2:500]  Ylog=off  Xlog=on  ShowGrid=off  save=off  variable=ZData  structure=0  ZoomFFT=off  StartTime=0.0  cycles=1  DisplayStyle=1  fundamental=60  FreqAxis=off  MaxFrequency=1000  frequencyindicesteady=1  RmsSteady=1  display=off
  send_sub2 : Outport
  wires:
  Three-Phase V-I Measurement2/2 -> Scope/2
  Three-Phase V-I Measurement2/1 -> Scope/1
  Three-Phase V-I Measurement3/2 -> [Iabc_tb], Mux/2  "Iabc_s"
  Mux/1 -> send_sub2/1
  Three-Phase V-I Measurement3/1 -> Mux/1  "Vabc_s"
  Three-Phase V-I Measurement1/1 -> Scope1/1, "abc -> dq (Power-Invariant)1"/1, To Workspace/1
  Three-Phase V-I Measurement1/2 -> Gain/1
  Discrete-Time Integrator/1 -> "abc -> dq (Power-Invariant)1"/2, "abc -> dq (Power-Invariant)"/2
  Constant/1 -> Discrete-Time Integrator/1
  "abc -> dq (Power-Invariant)1"/1 -> PQ Calculation (dq-Frame)/1
  "abc -> dq (Power-Invariant)"/1 -> PQ Calculation (dq-Frame)/2
  PQ Calculation (dq-Frame)/1 -> To Workspace2/1
  Sum4/1 -> Controlled Voltage Source2/1
  Demux/1 -> Fitted_Characteristic_Impedance1/1(In1)
  Propagation Function Compensation Subsystem/1(Out2) -> Sum3/2
  Fitted_Characteristic_Impedance1/2(Out3) -> Sum4/1
  Fitted_Characteristic_Impedance1/3(Out4) -> Sum5/1
  Demux1/6 -> Fitted_Characteristic_Impedance/3(In3)
  Propagation Function Compensation Subsystem/2(Out3) -> Sum4/2
  Sum5/1 -> Controlled Voltage Source6/1
  Fitted_Characteristic_Impedance/3(Out4) -> Sum/2
  Propagation Function Compensation Subsystem/3(Out4) -> Sum5/2
  Fitted_Characteristic_Impedance/2(Out3) -> Sum1/2
  Demux1/5 -> Fitted_Characteristic_Impedance/2(In2)
  Demux1/3 -> Sum/1
  Sum2/1 -> Propagation Function Compensation Subsystem/1(In1)
  Sum/1 -> Propagation Function Compensation Subsystem/3(In3)
  Sum1/1 -> Propagation Function Compensation Subsystem/2(In2)
  Demux/2 -> Fitted_Characteristic_Impedance1/2(In2)
  Demux1/1 -> Sum2/1
  Demux1/2 -> Sum1/1
  Sum3/1 -> Controlled Voltage Source1/1
  Fitted_Characteristic_Impedance1/1(Out2) -> Sum3/1
  Demux/3 -> Fitted_Characteristic_Impedance1/3(In3)
  Demux1/4 -> Fitted_Characteristic_Impedance/1(In1)
  Fitted_Characteristic_Impedance/1(Out2) -> Sum2/2
  receive_co/1 -> Demux1/1
  [Iabc_tb] -> Demux/1
  Gain/1 -> Scope1/2, "abc -> dq (Power-Invariant)"/1, To Workspace1/1
  connections:
  IBR1_GFM/RConn2 -- L1/LConn2 -- LOAD1/LConn2
  Three-Phase V-I Measurement3/LConn1 -- Distributed Parameters Line/LConn1
  Grid1/LConn1 -- Three-Phase V-I Measurement2/RConn1
  LOAD4/LConn1 -- R4/LConn1 -- Three-Phase V-I Measurement1/RConn1 -- L1/RConn1 -- L3/RConn1
  Three-Phase V-I Measurement2/LConn3 -- R4/RConn3
  L1/LConn1 -- IBR1_GFM/RConn1 -- LOAD1/LConn1
  L1/RConn2 -- R4/LConn2 -- Three-Phase V-I Measurement1/RConn2 -- LOAD4/LConn2 -- L3/RConn2
  Three-Phase V-I Measurement2/RConn2 -- Grid1/LConn2
  IBR1_GFM/RConn3 -- L1/LConn3 -- LOAD1/LConn3
  L1/RConn3 -- L3/RConn3 -- LOAD4/LConn3 -- Three-Phase V-I Measurement1/RConn3 -- R4/LConn3
  LOAD3/LConn1 -- IBR2_GFL/RConn1 -- L3/LConn1
  IBR2_GFL/RConn2 -- LOAD3/LConn2 -- L3/LConn2
  Three-Phase V-I Measurement2/RConn3 -- Grid1/LConn3
  Three-Phase V-I Measurement2/LConn1 -- R4/RConn1
  IBR2_GFL/RConn3 -- LOAD3/LConn3 -- L3/LConn3
  Three-Phase V-I Measurement2/LConn2 -- R4/RConn2
  Ground1/LConn1 -- Controlled Voltage Source1/LConn1 -- Controlled Voltage Source2/LConn1 -- Controlled Voltage Source6/LConn1
  Distributed Parameters Line/LConn2 -- Three-Phase V-I Measurement3/LConn2
  Three-Phase V-I Measurement3/LConn3 -- Distributed Parameters Line/LConn3
  R1/RConn1 -- Three-Phase V-I Measurement3/RConn1
  R1/RConn2 -- Three-Phase V-I Measurement3/RConn2
  R1/RConn3 -- Three-Phase V-I Measurement3/RConn3
  R1/LConn1 -- Controlled Voltage Source1/RConn1
  R1/LConn2 -- Controlled Voltage Source2/RConn1
  R1/LConn3 -- Controlled Voltage Source6/RConn1
  T_grid_0p38kV_66kV1/RConn1 -- Three-Phase V-I Measurement1/LConn1
  T_grid_0p38kV_66kV1/RConn2 -- Three-Phase V-I Measurement1/LConn2
  T_grid_0p38kV_66kV1/RConn3 -- Three-Phase V-I Measurement1/LConn3
  Distributed Parameters Line/RConn1 -- T_grid_0p38kV_66kV1/LConn1
  Distributed Parameters Line/RConn2 -- T_grid_0p38kV_66kV1/LConn2
  Distributed Parameters Line/RConn3 -- T_grid_0p38kV_66kV1/LConn3

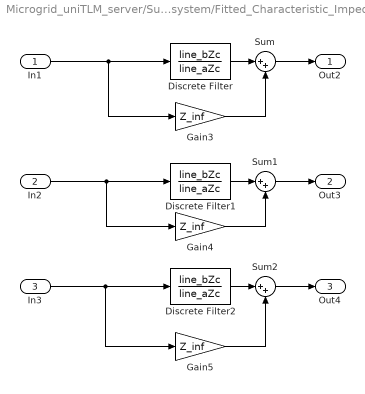
== system Microgrid_uniTLM_server/Subsystem/Fitted_Characteristic_Impedance ==
  In1 : Inport
  In2 : Inport  Port=2
  In3 : Inport  Port=3
  Discrete Filter : DiscreteFilter  LoadFcn=dspblkCoreblockFVToolHelper(gcbh,'load');  Numerator=line_bZc  Denominator=line_aZc
      settings: CopyFcn=dspblkCoreblockFVToolHelper(gcbh,'copy');  DeleteFcn=dspblkCoreblockFVToolHelper(gcbh,'close');  ModelCloseFcn=dspblkCoreblockFVToolHelper(gcbh,'close');  PreSaveFcn=dspblkCoreblockFVToolHelper(gcbh,'presave');  PostSaveFcn=dspblkCoreblockFVToolHelper(gcbh,'postsave');  CloseFcn=dspblkCoreblockFVToolHelper(gcbh,'close');
  Discrete Filter1 : DiscreteFilter  LoadFcn=dspblkCoreblockFVToolHelper(gcbh,'load');  Numerator=line_bZc  Denominator=line_aZc
      settings: CopyFcn=dspblkCoreblockFVToolHelper(gcbh,'copy');  DeleteFcn=dspblkCoreblockFVToolHelper(gcbh,'close');  ModelCloseFcn=dspblkCoreblockFVToolHelper(gcbh,'close');  PreSaveFcn=dspblkCoreblockFVToolHelper(gcbh,'presave');  PostSaveFcn=dspblkCoreblockFVToolHelper(gcbh,'postsave');  CloseFcn=dspblkCoreblockFVToolHelper(gcbh,'close');
  Discrete Filter2 : DiscreteFilter  LoadFcn=dspblkCoreblockFVToolHelper(gcbh,'load');  Numerator=line_bZc  Denominator=line_aZc
      settings: CopyFcn=dspblkCoreblockFVToolHelper(gcbh,'copy');  DeleteFcn=dspblkCoreblockFVToolHelper(gcbh,'close');  ModelCloseFcn=dspblkCoreblockFVToolHelper(gcbh,'close');  PreSaveFcn=dspblkCoreblockFVToolHelper(gcbh,'presave');  PostSaveFcn=dspblkCoreblockFVToolHelper(gcbh,'postsave');  CloseFcn=dspblkCoreblockFVToolHelper(gcbh,'close');
  Gain3 : Gain  Gain=Z_inf
  Gain4 : Gain  Gain=Z_inf
  Gain5 : Gain  Gain=Z_inf
  Sum : Sum  Inputs=|++
  Sum1 : Sum  Inputs=|++
  Sum2 : Sum  Inputs=|++
  Out2 : Outport
  Out3 : Outport  Port=2
  Out4 : Outport  Port=3
  wires:
  Sum1/1 -> Out3/1
  In3/1 -> Gain5/1, Discrete Filter2/1
  Discrete Filter2/1 -> Sum2/1
  Discrete Filter1/1 -> Sum1/1
  In2/1 -> Gain4/1, Discrete Filter1/1
  Discrete Filter/1 -> Sum/1
  In1/1 -> Gain3/1, Discrete Filter/1
  Sum/1 -> Out2/1
  Sum2/1 -> Out4/1
  Gain3/1 -> Sum/2
  Gain4/1 -> Sum1/2
  Gain5/1 -> Sum2/2

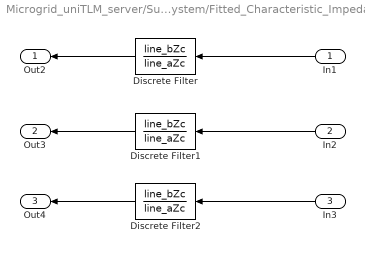
== system Microgrid_uniTLM_server/Subsystem/Fitted_Characteristic_Impedance1 ==
  In1 : Inport
  In2 : Inport  Port=2
  In3 : Inport  Port=3
  Discrete Filter : DiscreteFilter  LoadFcn=dspblkCoreblockFVToolHelper(gcbh,'load');  Numerator=line_bZc  Denominator=line_aZc
      settings: CopyFcn=dspblkCoreblockFVToolHelper(gcbh,'copy');  DeleteFcn=dspblkCoreblockFVToolHelper(gcbh,'close');  ModelCloseFcn=dspblkCoreblockFVToolHelper(gcbh,'close');  PreSaveFcn=dspblkCoreblockFVToolHelper(gcbh,'presave');  PostSaveFcn=dspblkCoreblockFVToolHelper(gcbh,'postsave');  CloseFcn=dspblkCoreblockFVToolHelper(gcbh,'close');
  Discrete Filter1 : DiscreteFilter  LoadFcn=dspblkCoreblockFVToolHelper(gcbh,'load');  Numerator=line_bZc  Denominator=line_aZc
      settings: CopyFcn=dspblkCoreblockFVToolHelper(gcbh,'copy');  DeleteFcn=dspblkCoreblockFVToolHelper(gcbh,'close');  ModelCloseFcn=dspblkCoreblockFVToolHelper(gcbh,'close');  PreSaveFcn=dspblkCoreblockFVToolHelper(gcbh,'presave');  PostSaveFcn=dspblkCoreblockFVToolHelper(gcbh,'postsave');  CloseFcn=dspblkCoreblockFVToolHelper(gcbh,'close');
  Discrete Filter2 : DiscreteFilter  LoadFcn=dspblkCoreblockFVToolHelper(gcbh,'load');  Numerator=line_bZc  Denominator=line_aZc
      settings: CopyFcn=dspblkCoreblockFVToolHelper(gcbh,'copy');  DeleteFcn=dspblkCoreblockFVToolHelper(gcbh,'close');  ModelCloseFcn=dspblkCoreblockFVToolHelper(gcbh,'close');  PreSaveFcn=dspblkCoreblockFVToolHelper(gcbh,'presave');  PostSaveFcn=dspblkCoreblockFVToolHelper(gcbh,'postsave');  CloseFcn=dspblkCoreblockFVToolHelper(gcbh,'close');
  Out2 : Outport
  Out3 : Outport  Port=2
  Out4 : Outport  Port=3
  wires:
  In1/1 -> Discrete Filter/1
  Discrete Filter/1 -> Out2/1
  In2/1 -> Discrete Filter1/1
  Discrete Filter1/1 -> Out3/1
  Discrete Filter2/1 -> Out4/1
  In3/1 -> Discrete Filter2/1

== system Microgrid_uniTLM_server/Subsystem/Grid1 ==
  Controlled Voltage Source1 : spsControlledVoltageSourceLib/Controlled Voltage Source  Initialize=on  Source_Type=AC  Amplitude=0  Phase=0  Frequency=0  Measurements=None
  Controlled Voltage Source2 : spsControlledVoltageSourceLib/Controlled Voltage Source  Initialize=on  Source_Type=AC  Amplitude=0  Phase=0  Frequency=0  Measurements=None
  Controlled Voltage Source6 : spsControlledVoltageSourceLib/Controlled Voltage Source  Initialize=on  Source_Type=AC  Amplitude=0  Phase=0  Frequency=0  Measurements=None
  Subsystem20 : Subsystem
  a : PMIOPort  Side=Left
  b : PMIOPort  Port=2  Side=Left
  c : PMIOPort  Port=3  Side=Left
  wires:
  Subsystem20/3(Ec) -> Controlled Voltage Source6/1
  Subsystem20/1(Ea) -> Controlled Voltage Source1/1
  Subsystem20/2(Eb) -> Controlled Voltage Source2/1
  connections:
  Controlled Voltage Source1/RConn1 -- a/RConn1
  Controlled Voltage Source6/RConn1 -- c/RConn1
  Controlled Voltage Source6/LConn1 -- Controlled Voltage Source2/LConn1 -- Controlled Voltage Source1/LConn1
  Controlled Voltage Source2/RConn1 -- b/RConn1
